simulink model "stateobsrv"  (R2015a)
settings: Solver=ode45  StartTime=0.0  StopTime=10.0  RelTol=1e-3
values from neighbouring files (symbols this model uses):
  A = [A, zeros(5,1); C(1,:), 0]    [L9_Q_opt.m]
  A8 = A - B*K - L*C    [L9.m]    (also in L9_Q_opt.m; Qe1.m; Qr1.m; Qr3.m)
  B = [B; 0]    [L9_Q_opt.m]
  B8 = L    [L9.m]    (also in L9_Q_opt.m; Qe1.m; Qr1.m; Qr3.m)
  C = [1 0 0 0 0 ... (first row only)    [L9.m]    (also in L9_Q_opt.m = [C, [0;0;0;0;0]; zeros(1,5), 0.00000000001]; Qe1.m; Qr1.m; Qr3.m)
  C8 = -K    [L9.m]    (also in L9_Q_opt.m; Qe1.m; Qr1.m; Qr3.m)
  D = [0 0 0 0 0]'    [L9.m]    (also in L9_Q_opt.m = [D; 0]; Qe1.m; Qr1.m; Qr3.m)
  D8 = [0 0 0 0 0]    [L9.m]    (also in L9_Q_opt.m = [0 0 0 0 0 0]; Qe1.m; Qr1.m; Qr3.m)
  x0 = [0 0 -0.005 0 0]'    [L9.m]    (also in L9_Q_opt.m = [0 0 -0.005 0 0, 0]'; Qe1.m = [0.01 0 0.01 0 0]'; Qr1.m; Qr3.m = [0.01 0 0.01 0 0]')
settings Model: Creator=afons  LastModifiedBy=afons

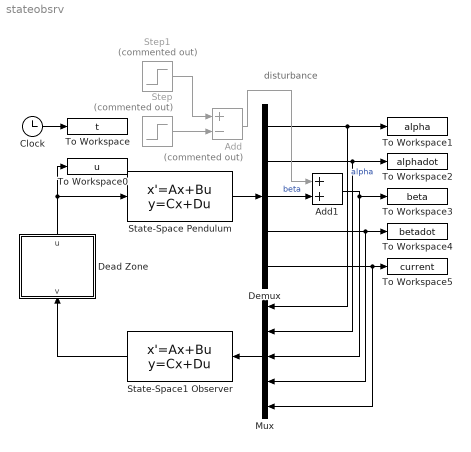
== system stateobsrv ==
  note: disturbance
  Add : Sum  Commented=on  Inputs=+-
  Add1 : Sum
  Clock : Clock
  Dead Zone : MATLAB Function  TreatAsAtomicUnit=on
  Demux : Demux  Outputs=5
  Mux : Mux  Inputs=5
  State-Space Pendulum : StateSpace  A=A  B=B  C=C  D=D  X0=x0
  State-Space1 Observer : StateSpace  A=A8  B=B8  C=C8  D=D8  X0=x0
  Step : Step  Commented=on  Time=1.1  After=0.3  SampleTime=0
  Step1 : Step  Commented=on  After=0.3  SampleTime=0
  To Workspace : ToWorkspace  VariableName=t  SampleTime=-1
  To Workspace0 : ToWorkspace  VariableName=u  SampleTime=-1
  To Workspace1 : ToWorkspace  VariableName=alpha  SampleTime=-1
  To Workspace2 : ToWorkspace  VariableName=alphadot  SampleTime=-1
  To Workspace3 : ToWorkspace  VariableName=beta  SampleTime=-1
  To Workspace4 : ToWorkspace  VariableName=betadot  SampleTime=-1
  To Workspace5 : ToWorkspace  VariableName=current  SampleTime=-1
  wires:
  State-Space Pendulum/1 -> Demux/1
  Clock/1 -> To Workspace/1
  Demux/3 -> Add1/2  "beta"
  Demux/1 -> Mux/1, To Workspace1/1  "alpha"
  Demux/2 -> Mux/2, To Workspace2/1
  Demux/5 -> Mux/5, To Workspace5/1
  Dead Zone/1(u) -> State-Space Pendulum/1, To Workspace0/1
  Step1/1 -> Add/1
  Step/1 -> Add/2
  Add/1 -> Add1/1
  Mux/1 -> State-Space1 Observer/1
  Add1/1 -> Mux/3, To Workspace3/1
  Demux/4 -> Mux/4, To Workspace4/1
  State-Space1 Observer/1 -> Dead Zone/1(v)

== matlab function stateobsrv/Dead Zone ==
  data: u output; v input
function u = dead_Zone(v)
%#codegen
if (abs(v) >= 0.32)
    u=v;
else
    u=0;
end;
